simulink model "crazyflie_full_model"  (R2018b)
settings: Solver=ode45  StartTime=0.0  StopTime=4.0  FixedStep=Ts  RelTol=1e-3
values from neighbouring files (symbols this model uses):
  Ts = 0.02    [main.m]
  yref = [yref states u]    [main.m]
  yref_e = states    [main.m]
undefined symbols (not defined in the file or in its folder): x0
settings Model: Creator=barbara  LastModifiedBy=barbara

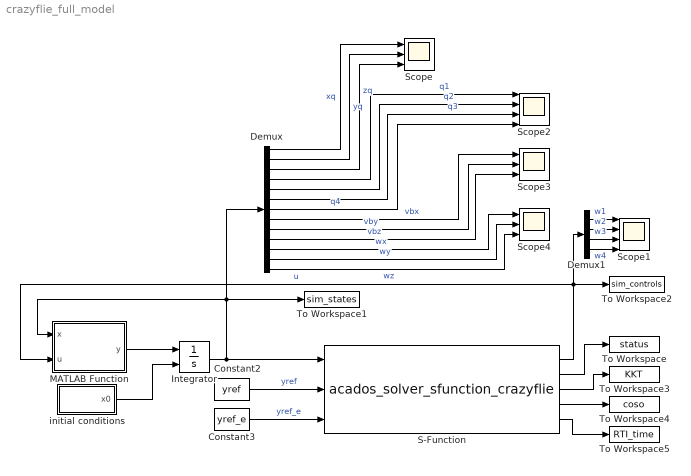
== system crazyflie_full_model ==
  Constant2 : Constant  Value=yref  SampleTime=Ts
  Constant3 : Constant  Value=yref_e  SampleTime=Ts
  Demux : Demux  Outputs=13
  Demux1 : Demux
  Integrator : Integrator  InitialConditionSource=external  InitialCondition=[1 0]'
  MATLAB Function : MATLAB Function  TreatAsAtomicUnit=on
  S-Function : S-Function  FunctionName=acados_solver_sfunction_crazyflie  SFunctionDeploymentMode=off  EnableBusSupport=off
  Scope : Scope  NumInputPorts=3
  Scope1 : Scope  NumInputPorts=4
  Scope2 : Scope  NumInputPorts=4
  Scope3 : Scope  NumInputPorts=3
  Scope4 : Scope  NumInputPorts=3
  To Workspace : ToWorkspace  VariableName=status  SaveFormat=Timeseries  SampleTime=Ts
  To Workspace1 : ToWorkspace  VariableName=sim_states  SaveFormat=Timeseries  SampleTime=Ts
  To Workspace2 : ToWorkspace  VariableName=sim_controls  SaveFormat=Timeseries  SampleTime=Ts
  To Workspace3 : ToWorkspace  VariableName=KKT  SaveFormat=Timeseries  SampleTime=Ts
  To Workspace4 : ToWorkspace  VariableName=coso  SaveFormat=Timeseries  SampleTime=Ts
  To Workspace5 : ToWorkspace  VariableName=RTI_time  SaveFormat=Timeseries  SampleTime=Ts
  initial conditions : Subsystem
      mask help: Edit <crazyflieData.m> for configuration.
      mask init:
      | crazyflieData
      mask Display: disp('x0')
  wires:
  MATLAB Function/1(y) -> Integrator/1
  S-Function/1 -> MATLAB Function/2(u), To Workspace2/1, Demux1/1  "u"
  S-Function/2 -> To Workspace/1
  S-Function/3 -> To Workspace3/1
  S-Function/4 -> To Workspace4/1
  S-Function/5 -> To Workspace5/1
  Constant2/1 -> S-Function/2  "yref"
  Constant3/1 -> S-Function/3  "yref_e"
  Demux/1 -> Scope/1  "xq"
  Demux/2 -> Scope/2  "yq"
  Demux/3 -> Scope/3  "zq"
  Demux/4 -> Scope2/1  "q1"
  Demux/5 -> Scope2/2  "q2"
  Demux/6 -> Scope2/3  "q3"
  Demux/7 -> Scope2/4  "q4"
  Demux/9 -> Scope3/2  "vby"
  Demux/10 -> Scope3/3  "vbz"
  Demux/8 -> Scope3/1  "vbx"
  Demux/11 -> Scope4/1  "wx"
  Demux/12 -> Scope4/2  "wy"
  Demux/13 -> Scope4/3  "wz"
  Demux1/1 -> Scope1/1  "w1"
  Demux1/2 -> Scope1/2  "w2"
  Demux1/3 -> Scope1/3  "w3"
  Demux1/4 -> Scope1/4  "w4"
  Integrator/1 -> S-Function/1, MATLAB Function/1(x), To Workspace1/1, Demux/1
  initial conditions/1(x0) -> Integrator/2

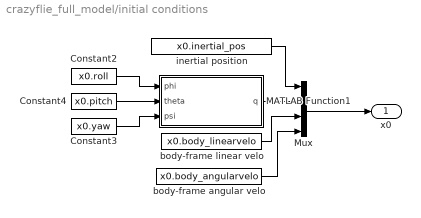
== system crazyflie_full_model/initial conditions ==
  Constant2 : Constant  Value=x0.roll  SampleTime=Ts
  Constant3 : Constant  Value=x0.yaw  SampleTime=Ts
  Constant4 : Constant  Value=x0.pitch  SampleTime=Ts
  MATLAB Function1 : MATLAB Function  TreatAsAtomicUnit=on
  Mux : Mux
  body-frame angular velo : Constant  Value=x0.body_angularvelo  VectorParams1D=off  SampleTime=Ts
  body-frame linear velo : Constant  Value=x0.body_linearvelo  SampleTime=Ts
  inertial position : Constant  Value=x0.inertial_pos  VectorParams1D=off  SampleTime=Ts
  x0 : Outport
  wires:
  Constant4/1 -> MATLAB Function1/2(theta)
  body-frame linear velo/1 -> Mux/3
  MATLAB Function1/1(q) -> Mux/2
  Mux/1 -> x0/1
  body-frame angular velo/1 -> Mux/4
  Constant3/1 -> MATLAB Function1/3(psi)
  inertial position/1 -> Mux/1
  Constant2/1 -> MATLAB Function1/1(phi)

== matlab function crazyflie_full_model/initial conditions/MATLAB Function1 ==
  data: phi input; theta input; q output; psi input
function q = euler2quatern(phi, theta, psi)
%EULER2QUATERN Converts a ZYX Euler angle orientation to a quaternion
%
%   q = euler2quatern(axis, angle)
%
%   Converts ZYX Euler angle orientation to a quaternion where phi is a
%   rotation around X, theta around Y and psi around Z.
%
%   For more information see:
%   http://x-io.co.uk/quaternions/
%
%	Date          Author          Notes
%	01/01/2015    SOH Madgwick    Initial release

    cosPsi = cos(psi * 0.5);
    sinPsi = sin(psi * 0.5);

    cosTheta = cos(theta * 0.5);
    sinTheta = sin(theta * 0.5);

    cosPhi = cos(phi * 0.5);
    sinPhi = sin(phi * 0.5);

    q = [cosPsi * cosTheta * cosPhi + sinPsi * sinTheta * sinPhi
         -(cosPsi * cosTheta * sinPhi - sinPsi * sinTheta * cosPhi)
         -(cosPsi * sinTheta * cosPhi + sinPsi * cosTheta * sinPhi)
         -(sinPsi * cosTheta * cosPhi - cosPsi * sinTheta * sinPhi)]; % must be conjugate
end

== matlab function crazyflie_full_model/MATLAB Function ==
  data: x input; u input; y output
function y = rhs(x,u)
%#codegen

g0 = 9.8;
mq  = 36.4e-3;
Ixx = 1.395e-5;
Iyy = 1.436e-5;
Izz = 2.173e-5;
Cd  = 7.9379e-12;
Ct  = 3.1582e-10;
dq  = 39.73e-3;


y = [  
        x(8)*(2*x(4)^2 + 2*x(5)^2 - 1) - x(9)*(2*x(4)*x(7) - 2*x(5)*x(6)) + x(10)*(2*x(4)*x(6) + 2*x(5)*x(7));
        x(9)*(2*x(4)^2 + 2*x(6)^2 - 1) + x(8)*(2*x(4)*x(7) + 2*x(5)*x(6)) - x(10)*(2*x(4)*x(5) - 2*x(6)*x(7));
        x(10)*(2*x(4)^2 + 2*x(7)^2 - 1) - x(8)*(2*x(4)*x(6) - 2*x(5)*x(7)) + x(9)*(2*x(4)*x(5) + 2*x(6)*x(7));
        - (x(5)*x(11))/2 - (x(6)*x(12))/2 - (x(7)*x(13))/2;
        (x(4)*x(11))/2 - (x(7)*x(12))/2 + (x(6)*x(13))/2;
        (x(7)*x(11))/2 + (x(4)*x(12))/2 - (x(5)*x(13))/2;
        (x(5)*x(12))/2 - (x(6)*x(11))/2 + (x(4)*x(13))/2;
        x(9)*x(13) - x(10)*x(12) - g0*(2*x(4)*x(6) - 2*x(5)*x(7));
        x(10)*x(11) - x(8)*x(13) + g0*(2*x(4)*x(5) + 2*x(6)*x(7));
        x(8)*x(12) - x(9)*x(11) + g0*(2*x(4)^2 + 2*x(7)^2 - 1) - (Ct*(u(1)^2 + u(2)^2 + u(3)^2 + u(4)^2))/mq;
        -(Ct*dq*(u(1)^2 + u(2)^2 - u(3)^2 - u(4)^2) - Iyy*x(12)*x(13) + Izz*x(12)*x(13))/Ixx;
        -(Ct*dq*(u(1)^2 - u(2)^2 - u(3)^2 + u(4)^2) - Ixx*x(11)*x(13) + Izz*x(11)*x(13))/Iyy;
        -(Cd*(u(1)^2 - u(2)^2 + u(3)^2 - u(4)^2) - Ixx*x(11)*x(12) + Iyy*x(11)*x(12))/Izz;
    ];
end
